simulink model "aufgabe1_sim"  (R2016b)
settings: Solver=VariableStepAuto  StartTime=0.0  StopTime=14  RelTol=1e-3
values from neighbouring files (symbols this model uses):
  ct = [0 0 1]    [aufgabe1.m]    (also in aufgabe2.m; aufgabe4.m; aufgabe5.m; aufgabe6.m = eye(3))
  g = 0.165707650406087    (= 0.165707650406)    [aufgabe2.m]
  gamma = dsys.B(:,1)    [aufgabe1.m]    (also in aufgabe6.m = dsys.B; aufgabe7.m = dsys.B)
  kt = [1.894974536721893,-0.520134683695267,0.478777536929102]    [aufgabe2.m]
  phi = dsys.A    [aufgabe1.m]    (also in aufgabe6.m; aufgabe7.m)
  Ta = 10e-03    (= 0.01)    [aufgabe1.m]    (also in aufgabe2.m; aufgabe4.m; aufgabe5.m; aufgabe6.m)
undefined symbols (not defined in the file or in its folder): DiscIntNeverNeededParam
libraries: cstblocks x2, simulink x1
settings Model: Creator=M  LastModifiedBy=M

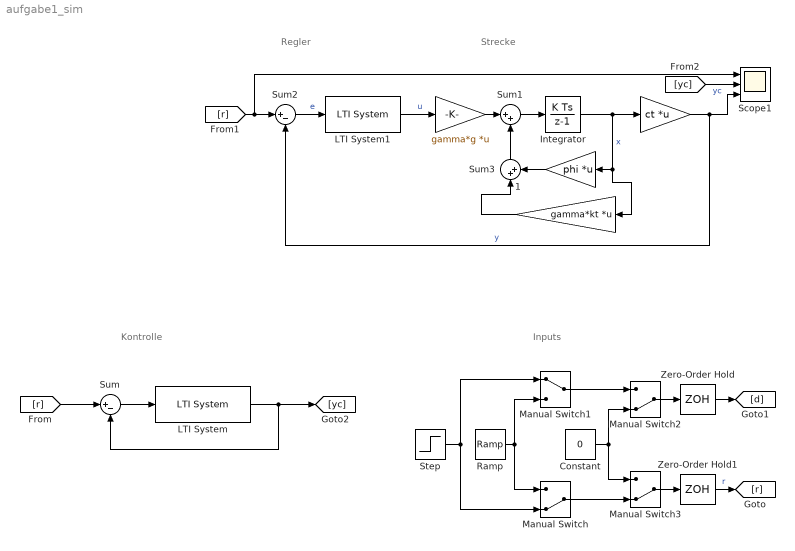
== system aufgabe1_sim ==
  note: Inputs
  note: Kontrolle
  note: Strecke
  note: Regler
  " " : Gain  Gain=phi  Multiplication=Matrix(K*u)
  "   " : Gain  Gain=ct  Multiplication=Matrix(K*u)
  "      " : Gain  Gain=gamma*g  Multiplication=Matrix(K*u)
  " 1" : Gain  Gain=gamma*kt  Multiplication=Matrix(K*u)
  Constant : Constant  Value=0
  Integrator : DiscreteIntegrator  InitialConditionSetting=State (most efficient)  SampleTime=Ta  ICPrevOutput=DiscIntNeverNeededParam  ICPrevScaledInput=DiscIntNeverNeededParam
  LTI System : cstblocks/LTI System  sys=Gz  IC=[]
  LTI System1 : cstblocks/LTI System  sys=tf(1,1)  IC=[]
  Manual Switch : ManualSwitch  CurrentSetting=0
  Manual Switch1 : ManualSwitch
  Manual Switch2 : ManualSwitch  CurrentSetting=0
  Manual Switch3 : ManualSwitch  CurrentSetting=0
  Ramp : simulink/Sources/Ramp  slope=1  start=1  X0=0
  Scope1 : Scope  NumInputPorts=3
  Step : Step  SampleTime=0
  Sum : Sum  Inputs=|+-
  Sum1 : Sum  Inputs=|++
  Sum2 : Sum  Inputs=|+-
  Sum3 : Sum  Inputs=|++
  Zero-Order Hold : ZeroOrderHold  SampleTime=-1
  Zero-Order Hold1 : ZeroOrderHold  SampleTime=-1
  wires:
  Manual Switch1/1 -> Manual Switch2/1
  Constant/1 -> Manual Switch3/1, Manual Switch2/2
  Manual Switch2/1 -> Zero-Order Hold/1
  Manual Switch3/1 -> Zero-Order Hold1/1
  Manual Switch/1 -> Manual Switch3/2
  Ramp/1 -> Manual Switch/1, Manual Switch1/2
  Step/1 -> Manual Switch/2, Manual Switch1/1
  Sum/1 -> LTI System/1
  LTI System/1 -> [yc], Sum/2
  Zero-Order Hold1/1 -> [r]  "r"
  Zero-Order Hold/1 -> [d]
  Integrator/1 -> " 1"/1, " "/1, "   "/1  "x"
  Sum1/1 -> Integrator/1
  "      "/1 -> Sum1/1
  [r] -> Sum2/1, Scope1/1
  [r] -> Sum/1
  [yc] -> Scope1/2  "yc"
  "   "/1 -> Scope1/3, Sum2/2  "y"
  Sum2/1 -> LTI System1/1  "e"
  LTI System1/1 -> "      "/1  "u"
  " "/1 -> Sum3/2
  Sum3/1 -> Sum1/2
  " 1"/1 -> Sum3/1
